simulink model "SegheriaSCADA2"  (R2024b)
settings: Solver=FixedStepAuto  StartTime=0.0  StopTime=60  FixedStep=0.001  RelTol=1e-3
values from neighbouring files (symbols this model uses):
  b = t + 2*s    (= 3.6)    [ParametriSegheria.m]    (also in ParametriSegheriaDinamica.m)
  h = 70    [ParametriSegheria.m]
  i_id = 60    [ParametriSegheria.m]
  kc = [0 35 40 50 55 90]    [ParametriSegheria.m]    (also in ParametriSegheriaDinamica.m = [0, 25, 30, 35, 50, 70])
  Kt = 2    [ParametriSegheria.m]    (also in ParametriSegheriaDinamica.m = 10000)
  Lt = 4    [ParametriSegheria.m]    (also in ParametriSegheriaDinamica.m)
  Mag_D = [0 430 320 260 230 540]    [ParametriSegheria.m]    (also in ParametriSegheriaDinamica.m = [0 randi([220 500], 1, 150)])
  Mag_legno = [0 1 5 2 4 3]    [ParametriSegheria.m]    (also in ParametriSegheriaDinamica.m = [0 randi([1 5], 1, 150)])
  omega = 50    [ParametriSegheria.m]
  SR = Rs/Rm    (= 5.33333333333)    [ParametriSegheria.m]    (also in ParametriSegheriaDinamica.m)
  Tloss = Tatt+ Tdamp    (= 17.3333333333)    [ParametriSegheria.m]
undefined symbols (not defined in the file or in its folder): i_max
libraries: slpidlib x1, simulink x1
settings Model: Creator=samue  LastModifiedBy=samue

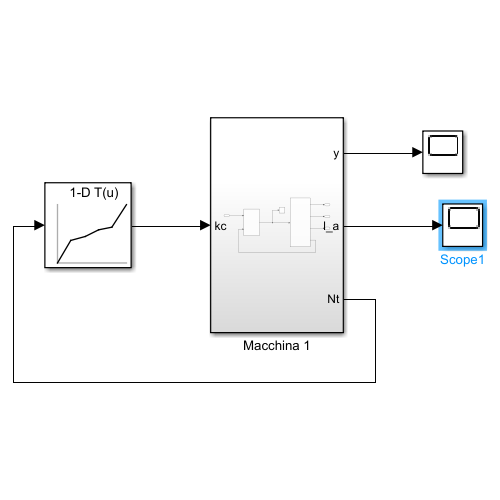
[thumbnail: Simulink's stored preview of the top-level diagram]
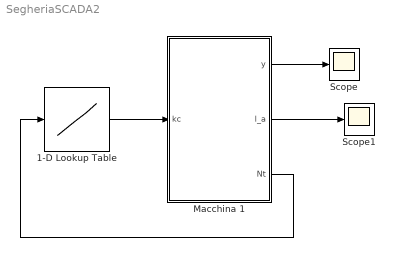
== system SegheriaSCADA2 ==
  1-D Lookup Table : Lookup_n-D  NumberOfTableDimensions=1  BreakpointsForDimension1=[0 1 2 3 4 5 ]  Table=kc  InternalRulePriority=Speed  RndMeth=Simplest
  Macchina 1 : Subsystem
  Scope : Scope
  Scope1 : Scope
  wires:
  Macchina 1/3(Nt) -> 1-D Lookup Table/1
  1-D Lookup Table/1 -> Macchina 1/1(kc)
  Macchina 1/1(y) -> Scope/1
  Macchina 1/2(l_a) -> Scope1/1

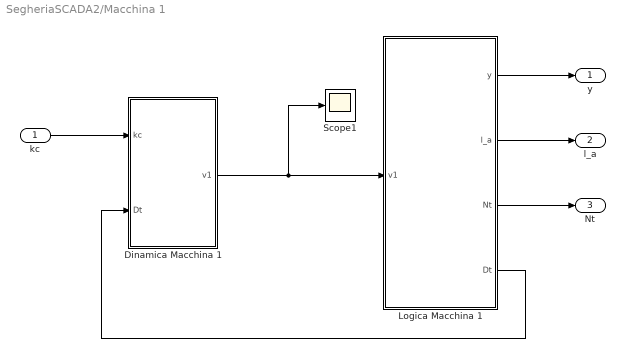
== system SegheriaSCADA2/Macchina 1 ==
  kc : Inport
  Dinamica Macchina 1 : Subsystem
  Logica Macchina 1 : Subsystem
  Scope1 : Scope
  y : Outport
  l_a : Outport  Port=2
  Nt : Outport  Port=3
  wires:
  kc/1 -> Dinamica Macchina 1/1(kc)
  Dinamica Macchina 1/1(v1) -> Scope1/1, Logica Macchina 1/1(v1)
  Logica Macchina 1/3(Nt) -> Nt/1
  Logica Macchina 1/4(Dt) -> Dinamica Macchina 1/2(Dt)
  Logica Macchina 1/1(y) -> y/1
  Logica Macchina 1/2(l_a) -> l_a/1

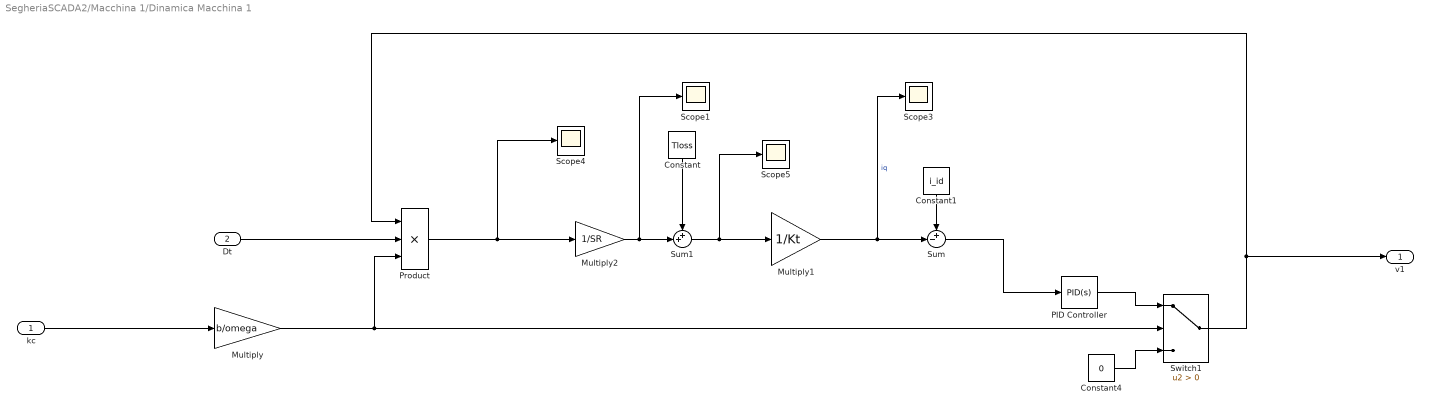
== system SegheriaSCADA2/Macchina 1/Dinamica Macchina 1 ==
  kc : Inport
  Dt : Inport  Port=2
  Constant : Constant  Value=Tloss
  Constant1 : Constant  Value=i_id
  Constant4 : Constant  Value=0
  Multiply : Gain  Gain=b/omega
  Multiply1 : Gain  Gain=1/Kt
  Multiply2 : Gain  Gain=1/SR
  PID Controller : slpidlib/PID Controller  Controller=PID  Form=Parallel  TimeDomain=Continuous-time  UseExternalTs=off  SampleTime=-1  IntegratorMethod=Forward Euler  FilterMethod=Forward Euler  ControllerParametersSource=internal  P=0  I=0.0048685791703887  UseKiTs=off  D=0  UseExternalDerivativeSource=off  N=100  UseFilter=on  TunerSelectOption=Transfer Function Based (PID Tuner App)  InitialConditionSource=internal  InitialConditionForIntegrator=0  InitialConditionForFilter=0  DifferentiatorICPrevScaledInput=0  ExternalReset=none  TrackingMode=off  Kt=1  LimitOutput=off  SatLimitsSource=internal  UpperSaturationLimit=i_max  LowerSaturationLimit=-inf  LinearizeAsGain=on  AntiWindupMode=none  Kb=1  LimitIntegrator=off  UpperIntegratorSaturationLimit=inf  LowerIntegratorSaturationLimit=-inf  POutMin=[]  POutMax=[]  IOutMin=[]  IOutMax=[]  DOutMin=[]  DOutMax=[]  NOutMin=[]  NOutMax=[]  SumOutMin=[]  SumOutMax=[]  SaturationOutMin=[]  SaturationOutMax=[]  PParamMin=[]  PParamMax=[]  IParamMin=[]  IParamMax=[]  DParamMin=[]  DParamMax=[]  NParamMin=[]  NParamMax=[]  KbParamMin=[]  KbParamMax=[]  KtParamMin=[]  KtParamMax=[]  KbOutMin=[]  KbOutMax=[]  KtOutMin=[]  KtOutMax=[]  IntegratorOutMin=[]  IntegratorOutMax=[]  FilterOutMin=[]  FilterOutMax=[]  SumI1OutMin=[]  SumI1OutMax=[]  SumI2OutMin=[]  SumI2OutMax=[]  SumI3OutMin=[]  SumI3OutMax=[]  SumI4OutMin=[]  SumI4OutMax=[]  SumDOutMin=[]  SumDOutMax=[]  DifferentiatorOutMin=[]  DifferentiatorOutMax=[]  FilterDiffOutCoefMin=[]  FilterDiffOutCoefMax=[]  ReciprocalOutMin=[]  ReciprocalOutMax=[]  SumDenOutMin=[]  SumDenOutMax=[]  SumNumOutMin=[]  SumNumOutMax=[]  DivideOutMin=[]  DivideOutMax=[]  UdiffTsProdOutMin=[]  UdiffTsProdOutMax=[]  NTsProdOutMin=[]  NTsProdOutMax=[]  UintegralTsProdOutMin=[]  UintegralTsProdOutMax=[]  UngainTsProdOutMin=[]  UngainTsProdOutMax=[]  ClampingZeroOutDataTypeStr=Inherit: Inherit via back propagation  ClampingZeroOutMin=[]  ClampingZeroOutMax=[]  FilterDenConstantOutDataTypeStr=Inherit: Inherit via back propagation  FilterDenConstantOutMin=[]  FilterDenConstantOutMax=[]  PCopyOutDataTypeStr=Inherit: Inherit via back propagation  PCopyOutMin=[]  PCopyOutMax=[]  NCopyOutDataTypeStr=Inherit: Inherit via back propagation  NCopyOutMin=[]  NCopyOutMax=[]  IntegratorContinuousStateAttributes=''  IntegratorStateMustResolveToSignalObject=off  IntegratorRTWStateStorageClass=Auto  FilterContinuousStateAttributes=''  FilterStateMustResolveToSignalObject=off  FilterRTWStateStorageClass=Auto  ParallelPVariant=InternalParameters  IdealPVariant=Disabled  IVariant=InternalParameters  DVariant=InternalParameters  IntegratorVariant=Continuous  SatVariant=Disabled  AWVariant=Passthrough  PCopyVariant=Disabled  TRVariant=Disabled  FdbkBlocksVariant=Forward  IdealPFdbkVariant=Disabled  SatFdbkVariant=Disabled  DerivativeFilterVariant=ContFilter  NVariant=InternalParameters  NCopyVariant=Disabled  FilterICVariant=InternalICsFilter  IntegratorICVariant=InternalICs  ExternalResetVariant=Disabled  TRSumVariant=Passthrough  SumFdbkVariant=Disabled  SumVariant=Sum_PID  TsampFilterVariant=InternalTs  TsampNgainVariant=Passthrough  TsampIntegralVariant=Disabled_SignalSpec  ExternalSaturationOutDataTypeStr=Inherit: Same as second input  DerivativeSourceVariant=ErrorSignal  PreIntVariant=InternalPreInt
  Product : Product  Inputs=3
  Scope{1,3..5} (4 alike) : Scope
  Sum : Sum  Inputs=+-|
  Sum1 : Sum  Inputs=++|
  Switch1 : Switch  Criteria=u2 > Threshold  SaturateOnIntegerOverflow=off  InputSameDT=off
  v1 : Outport
  wires:
  Constant4/1 -> Switch1/3
  Product/1 -> Scope4/1, Multiply2/1
  PID Controller/1 -> Switch1/1
  Multiply1/1 -> Scope3/1, Sum/2  "iq"
  Multiply/1 -> Product/3, Switch1/2
  kc/1 -> Multiply/1
  Switch1/1 -> v1/1, Product/1
  Constant1/1 -> Sum/1
  Sum/1 -> PID Controller/1
  Multiply2/1 -> Scope1/1, Sum1/2
  Sum1/1 -> Scope5/1, Multiply1/1
  Constant/1 -> Sum1/1
  Dt/1 -> Product/2

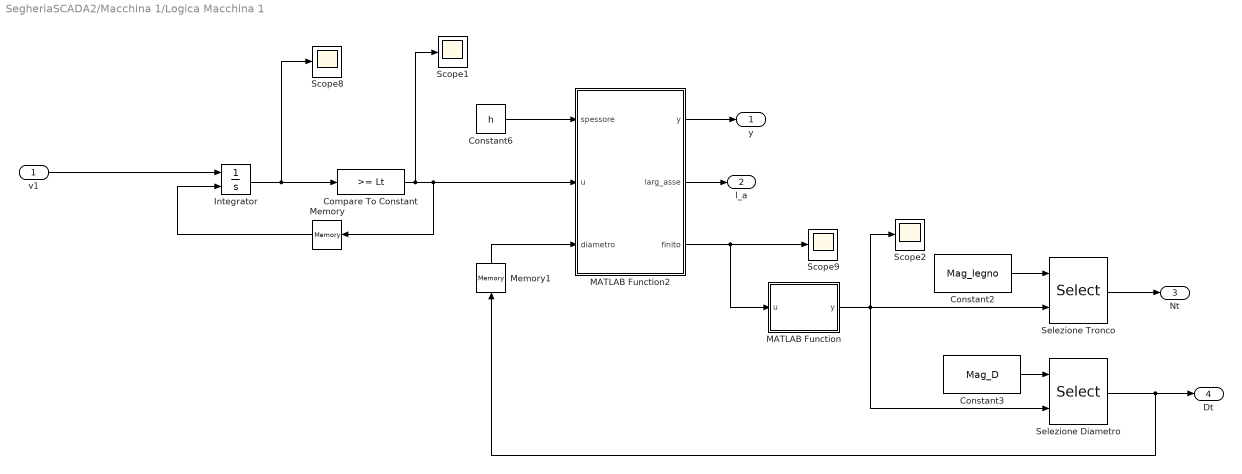
== system SegheriaSCADA2/Macchina 1/Logica Macchina 1 ==
  v1 : Inport
  Compare To Constant : simulink/Logic and Bit Operations/Compare To Constant  relop=>=  const=Lt  OutDataTypeStr=boolean
  Constant2 : Constant  Value=Mag_legno
  Constant3 : Constant  Value=Mag_D
  Constant6 : Constant  Value=h
  Integrator : Integrator  ExternalReset=rising
  MATLAB Function : MATLAB Function  TreatAsAtomicUnit=on
  MATLAB Function2 : MATLAB Function  TreatAsAtomicUnit=on
  Memory : Memory
  Memory1 : Memory
  Scope{1..2,8..9} (4 alike) : Scope
  Selezione Diametro : Selector  IndexMode=Zero-based  InputPortWidth=length(Mag_D)  IndexOptions=Index vector (port)  Indices=[1 3]  OutputSizes=1
  Selezione Tronco : Selector  IndexMode=Zero-based  InputPortWidth=length(Mag_legno)  IndexOptions=Index vector (port)  Indices=[1 3]  OutputSizes=1
  y : Outport
  l_a : Outport  Port=2
  Nt : Outport  Port=3
  Dt : Outport  Port=4
  wires:
  Constant6/1 -> MATLAB Function2/1(spessore)
  Selezione Diametro/1 -> Dt/1, Memory1/1
  MATLAB Function2/3(finito) -> Scope9/1, MATLAB Function/1(u)
  Memory/1 -> Integrator/2
  Memory1/1 -> MATLAB Function2/3(diametro)
  Constant2/1 -> Selezione Tronco/1
  v1/1 -> Integrator/1
  Integrator/1 -> Compare To Constant/1, Scope8/1
  Constant3/1 -> Selezione Diametro/1
  MATLAB Function/1(y) -> Selezione Diametro/2, Scope2/1, Selezione Tronco/2
  MATLAB Function2/1(y) -> y/1
  Selezione Tronco/1 -> Nt/1
  MATLAB Function2/2(larg_asse) -> l_a/1
  Compare To Constant/1 -> Scope1/1, Memory/1, MATLAB Function2/2(u)

== matlab function SegheriaSCADA2/Macchina 1/Logica Macchina 1/MATLAB Function ==
  data: u input; y output; Mag_legno parameter
function y = fcn(u, Mag_legno)
    persistent counter
    if isempty(counter)
        counter = 1;
    end

    if u == 1
        counter = counter + 1;
    end

    y = counter;
    
    if y > length(Mag_legno)-1
        y = 0;
    end

end

== matlab function SegheriaSCADA2/Macchina 1/Logica Macchina 1/MATLAB Function2 ==
  settings: updateMethod=DISCRETE
  data: spessore input; u input; y output; larg_asse output; finito output; diametro input
function [y, larg_asse, finito]= fcn(spessore, u, diametro)
    persistent counter 

    max_assi = floor(diametro / spessore);
    finito = 0;
    

    if isempty(counter)
        counter = 0;
    end

    % Conto assi tagliate
    if u == 1
        counter = counter + 1;
    end

    % Quando finisco tronco segnalo e azzero counter
    if counter > max_assi
        finito = 1;
        counter = 0;
    end

    % Calcolo larghezza delle assi
    distanza_bordo = counter * spessore;
    h = abs(diametro/2 - distanza_bordo + (spessore/2));
    
    if counter == 0
        larg_asse = 0;
    else
        larg_asse = 2 * sqrt((diametro/2)^2-h^2);
    end

    y = counter;
end
